simulink model "ultra_slow_plant"  (R2015a)
settings: Solver=ode45  StartTime=0.0  StopTime=14000  RelTol=1e-3
settings Model: Creator=ra428  LastModifiedBy=ra428

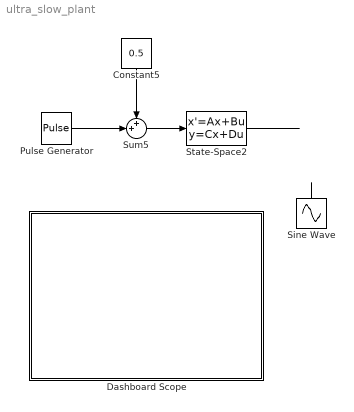
== system ultra_slow_plant ==
  Constant5 : Constant  Value=0.5
  Dashboard Scope : Subsystem  DialogController=hmiCreateDDGDialog  IsWebBlock=on  mask(MathWorksWebBlock){webBlockId=d36c273f-0639-4b36-8f7a-aa8a1bb7231a, webBlockType=sdiscope, ShowInitialText=on, HMISrcModelName=untitled}
      mask prompts: webBlockId "WebBlock Id"; webBlockType "WebBlock Type"; HMISrcModelName "Source Model"
      mask Help: helpview([docroot '/mapfiles/simulink.map'], 'hmi_scope')
      mask Display:
      | if strcmp(get_param(bdroot(gcb),'BlockDiagramType'), 'library')
      |     image([(matlabroot) '/toolbox/simulink/hmi/icons/DashboardScope.png']);
      | end
  Pulse Generator : DiscretePulseGenerator  PulseType=Time based  Amplitude=-1  Period=6000  PulseWidth=50
  Sine Wave : Sin  Amplitude=.25  Frequency=.001  SampleTime=0
  State-Space2 : StateSpace  A=-1/1500  B=-1/1500  D=0  X0=-.2
  Sum5 : Sum  Inputs=++|
  wires:
  Pulse Generator/1 -> Sum5/2
  Sum5/1 -> State-Space2/1
  Constant5/1 -> Sum5/1
  State-Space2/1 -> ?
  Sine Wave/1 -> ?

== system ultra_slow_plant/Dashboard Scope ==
